simulink model "ce4951transmitter"  (R2020b)
settings: Solver=VariableStepAuto  StartTime=0.0  StopTime=32  RelTol=1e-3
libraries: simulink_extras x8, dspsrcs4 x1
settings Model: Creator=Andy  LastModifiedBy=Andy

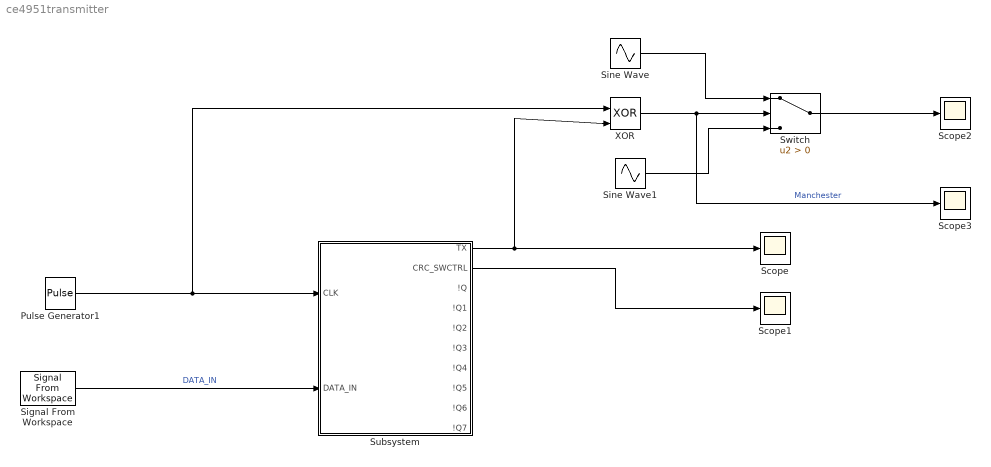
== system ce4951transmitter ==
  Pulse Generator1 : DiscretePulseGenerator  PulseType=Time based  Period=1  PulseWidth=50
  Scope{,1..3} (4 alike) : Scope
  Signal From Workspace : dspsrcs4/Signal From Workspace  X=[0 1 0 0 0 0 0 1 0 1 0 0 0 0 1 0 0 1 0 0 0 0 1 1 0 0 0 0 0 0 0 0]  Ts=1  nsamps=1  OutputAfterFinalValue=Setting to zero  ignoreOrWarnInputAndFrameLengths=off  OutputFrames=off
  Sine Wave : Sin  Frequency=2*pi*2  SampleTime=0
  Sine Wave1 : Sin  Frequency=2*pi*4  SampleTime=0
  Subsystem : Subsystem
  Switch : Switch  Criteria=u2 > Threshold
  XOR : Logic  Operator=XOR  IconShape=distinctive  AllPortsSameDT=off  OutDataTypeStr=boolean
  wires:
  Pulse Generator1/1 -> XOR/1, Subsystem/1(CLK)
  Signal From Workspace/1 -> Subsystem/2(DATA_IN)  "DATA_IN"
  Subsystem/1(TX) -> XOR/2, Scope/1
  Subsystem/2(CRC_SWCTRL) -> Scope1/1
  XOR/1 -> Scope3/1, Switch/2  "Manchester"
  Sine Wave/1 -> Switch/1
  Sine Wave1/1 -> Switch/3
  Switch/1 -> Scope2/1

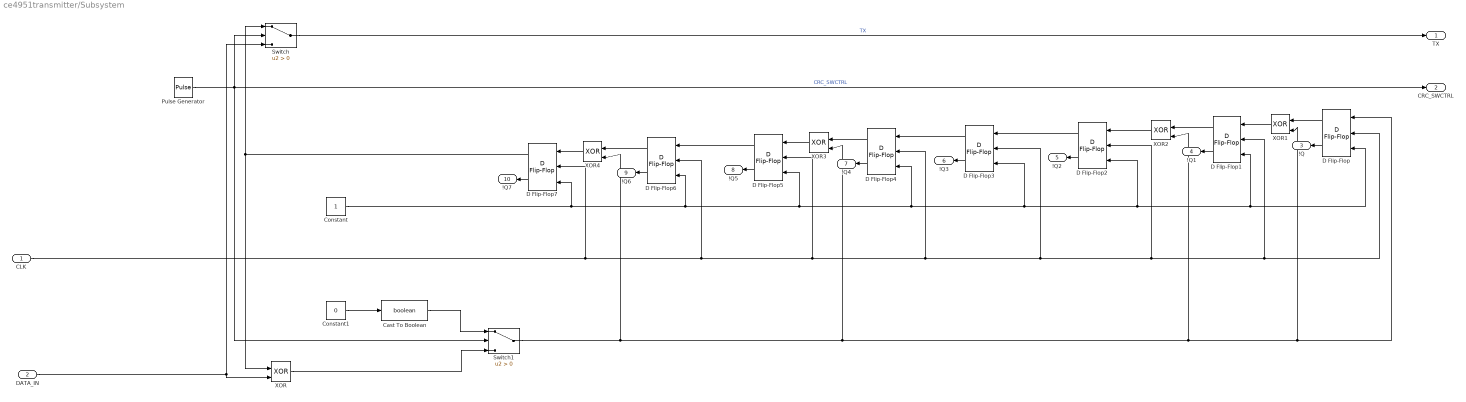
== system ce4951transmitter/Subsystem ==
  CLK : Inport
  DATA_IN : Inport  Port=2
  Cast To Boolean : DataTypeConversion  OutDataTypeStr=boolean
  Constant : Constant
  Constant1 : Constant  Value=0
  D Flip-Flop{,1..7} (8 alike) : simulink_extras/Flip Flops/D Flip-Flop
  Pulse Generator : DiscretePulseGenerator  PulseType=Time based  Period=32  PulseWidth=25  PhaseDelay=24
  Switch : Switch  Criteria=u2 > Threshold
  Switch1 : Switch  Criteria=u2 > Threshold
  XOR{,1..4} (5 alike) : Logic  Operator=XOR  IconShape=distinctive  AllPortsSameDT=off  OutDataTypeStr=boolean
  TX : Outport
  CRC_SWCTRL : Outport  Port=2
  !Q : Outport  Port=3
  !Q1 : Outport  Port=4
  !Q2 : Outport  Port=5
  !Q3 : Outport  Port=6
  !Q4 : Outport  Port=7
  !Q5 : Outport  Port=8
  !Q6 : Outport  Port=9
  !Q7 : Outport  Port=10
  wires:
  XOR1/1 -> D Flip-Flop1/1
  D Flip-Flop2/2 -> !Q2/1
  Constant1/1 -> Cast To Boolean/1
  D Flip-Flop4/2 -> !Q4/1
  CLK/1 -> D Flip-Flop6/2, D Flip-Flop5/2, D Flip-Flop4/2, D Flip-Flop3/2, D Flip-Flop2/2, D Flip-Flop1/2, D Flip-Flop/2, D Flip-Flop7/2
  D Flip-Flop7/1 -> Switch/1, XOR/1
  D Flip-Flop1/1 -> XOR2/1
  Constant/1 -> D Flip-Flop5/3, D Flip-Flop4/3, D Flip-Flop3/3, D Flip-Flop2/3, D Flip-Flop1/3, D Flip-Flop/3, D Flip-Flop6/3, D Flip-Flop7/3
  Switch/1 -> TX/1  "TX"
  D Flip-Flop5/1 -> D Flip-Flop6/1
  Switch1/1 -> XOR4/2, XOR2/2, XOR1/2, D Flip-Flop/1, XOR3/2
  Pulse Generator/1 -> CRC_SWCTRL/1, Switch1/2, Switch/2  "CRC_SWCTRL"
  XOR2/1 -> D Flip-Flop2/1
  XOR3/1 -> D Flip-Flop5/1
  D Flip-Flop6/2 -> !Q6/1
  DATA_IN/1 -> Switch/3, XOR/2
  D Flip-Flop3/1 -> D Flip-Flop4/1
  D Flip-Flop5/2 -> !Q5/1
  Cast To Boolean/1 -> Switch1/1
  D Flip-Flop2/1 -> D Flip-Flop3/1
  D Flip-Flop/1 -> XOR1/1
  XOR/1 -> Switch1/3
  D Flip-Flop4/1 -> XOR3/1
  D Flip-Flop3/2 -> !Q3/1
  D Flip-Flop6/1 -> XOR4/1
  D Flip-Flop/2 -> !Q/1
  XOR4/1 -> D Flip-Flop7/1
  D Flip-Flop7/2 -> !Q7/1
  D Flip-Flop1/2 -> !Q1/1
